simulink model "example_Storage_type3conf"  (R2016b)
settings: Solver=ode45  StartTime=0.0  StopTime=3*3600-2  RelTol=1e-3  EnableMultiTasking=on
undefined symbols (not defined in the file): path_carnot
libraries: carnot x12, simulink x3
settings Model: Creator=drhf  LastModifiedBy=drhf
settings DataIOCC: LimitDataPoints=on  SaveFormat=Array
settings OptimizationCC: ExpressionDepthLimit=2147483647  LifeSpan=inf
settings DebuggingCC: UnderspecifiedInitializationDetection=Classic  MergeDetectMultiDrivingBlocksExec=none  SolverPrmCheckMsg=warning  StateNameClashWarn=warning  SFUnexpectedBacktrackingDiag=warning  SFNoUnconditionalDefaultTransitionDiag=warning  SFExecutionAtInitializationDiag=none
settings HardwareCC: ProdBitPerPointer=32  ProdBitPerSizeT=32  ProdBitPerPtrDiffT=32  ProdLargestAtomicFloat=None  ProdIntDivRoundTo=Undefined  ProdEndianess=Unspecified  ProdWordSize=32  ProdHWDeviceType=32-bit Generic
settings ModelReferenceCC: PropagateSignalLabelsOutOfModel=off
settings GRTTargetCC: TargetLangStandard=C89/C90 (ANSI)  GeneratePreprocessorConditionals=Disable all  CombineOutputUpdateFcns=off  GRTInterface=on
settings ConfigComp: CovMetricSettings=dw  CovHtmlReporting=on  CovSaveCumulativeToWorkspaceVar=on  CovSaveSingleToWorkspaceVar=on  CovExternalEMLEnable=off

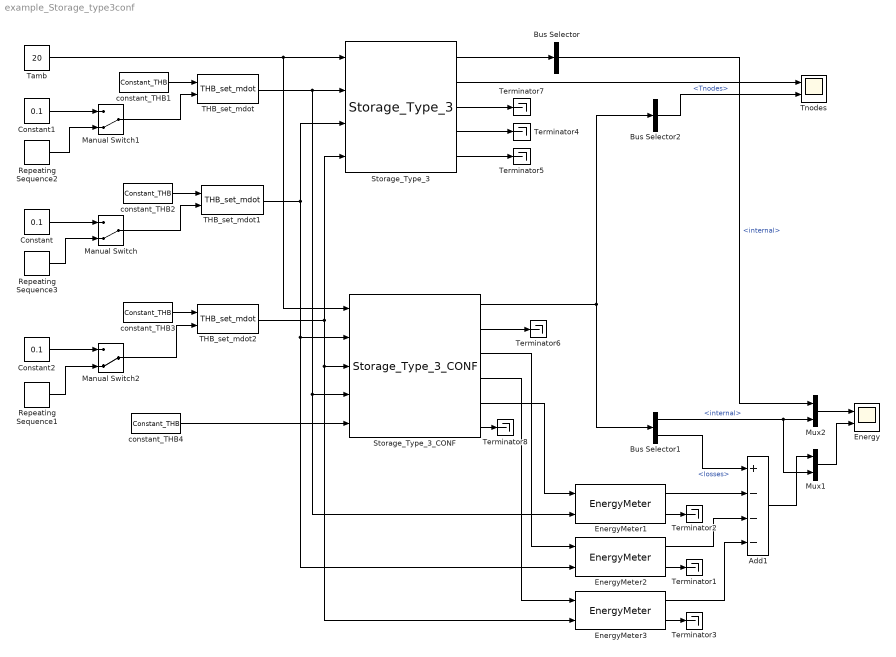
== system example_Storage_type3conf ==
  Add1 : Sum  Inputs=+---
  Bus Selector : BusSelector  OutputSignals=energy.internal
  Bus Selector1 : BusSelector  OutputSignals=energy.internal,energy.losses
  Bus Selector2 : BusSelector  OutputSignals=Tnodes
  Constant : Constant  Value=0.1
  Constant1 : Constant  Value=0.1
  Constant2 : Constant  Value=0.1
  Energy : Scope  NumInputPorts=2
  EnergyMeter1 : carnot/Control/EnergyMeter
  EnergyMeter2 : carnot/Control/EnergyMeter
  EnergyMeter3 : carnot/Control/EnergyMeter
  Manual Switch : ManualSwitch  CurrentSetting=0
  Manual Switch1 : ManualSwitch  CurrentSetting=0
  Manual Switch2 : ManualSwitch  CurrentSetting=0
  Mux1 : Mux  Inputs=2
  Mux2 : Mux  Inputs=2
  Repeating Sequence1 : simulink/Sources/Repeating Sequence  rep_seq_t=[ 0 3600 3600+eps(3600) 7200 7200+eps(7200) 10800]  rep_seq_y=[ 0.12 0.12 0.11+0*eps(3600) 0.11 0.05+0*eps(7200) 0.05]
  Repeating Sequence2 : simulink/Sources/Repeating Sequence  rep_seq_t=[ 0 3600 3600+eps(3600) 7200 7200+eps(7200) 10440 10440+eps(10440) 11160]  rep_seq_y=[ 0 0 0.05+0*eps(3600) 0.05 0.2+0*eps(7200) 0.2 0+0*eps(10440) 0]
  Repeating Sequence3 : simulink/Sources/Repeating Sequence  rep_seq_t=[ 0 3600 3600+eps(3600) 7200 7200+eps(7200) 10800]  rep_seq_y=[ 0 0 0.1+0*eps(3600) 0.1 0.15+0*eps(7200) 0.15]
  Storage_Type_3 : carnot/Storage/Thermal/Storage_Type_3  uloss=1  ubot=1  utop=1  cond=1  volume=0.3  dia=0.5  pos=standing cylinder  h_in_hxup=0.81  h_out_hxup=0.56  ua0_hxup=80  uam_hxup=0.2  uat_hxup=0.5  dplin_hxup=100  dpqua_hxup=100  h_in_hxlw=0.48  h_out_hxlw=0.04  ua0_hxlw=100  uam_hxlw=0.2  uat_hxlw=0.5  dplin_hxlw=100  dpqua_hxlw=100  h_in=0  h_out=1  diapipe=0.04  t0=[10:5:55]  nodes=10  mpoints=10
  Storage_Type_3_CONF : carnot/Storage/Thermal/Storage_Type_3_CONF  t0=[10:5:55]  hgt=1.5279  stgtype=3  tini=[10 15 20 25 30 35 40 45 50 55]  mpts=[1 2 3 4 5 6 7 8 9 10]  PathName=fullfile(path_carnot('libsl'),'Storage','Thermal','Storage_Type_3_CONF','parameter_set')  FileName='StorageType3_300_L.mat'  userPath=off  userParam=off  uwall=1  ubot=1  utop=1  axcond=1  volume=0.3  dia=0.5  standing=standing cylinder  nodes=10  mpoints=10  Tsensor=[0.1 0.5 0.7]  hx1inlet=0.8  hx1outlet=0.6  hx1dia=0.03  hx1uac=50  hx1uam=0.15  hx1uat=0.6  hx1dpqua=20  hx1dplin=20  hx2inlet=0.4  hx2outlet=0  hx2dia=0.03  hx2uac=100  hx2uam=0.15  hx2uat=0.6  hx2dplin=30  hx2dpqua=30  pipe1inlet=0  pipe1outlet=1  pipe1dia=0.03  pipe2inlet=0.6  pipe2outlet=1  pipe2dia=0.03
  THB_set_mdot : carnot/Source/Simple/THB_set_mdot
  THB_set_mdot1 : carnot/Source/Simple/THB_set_mdot
  THB_set_mdot2 : carnot/Source/Simple/THB_set_mdot
  Tamb : Constant  Value=20
  Terminator{1..8} (8 alike) : Terminator
  Tnodes : Scope  NumInputPorts=2
  constant_THB1 : carnot/Source/Simple/Constant_THB  t=10  mdot=0*100/3600  p=1e5  mID=Full Pressure Drop with Static Height  fluid=Water  mix=0  mix2=0  mix3=0  dia=0.02  hgt=0
  constant_THB2 : carnot/Source/Simple/Constant_THB  t=55  mdot=0*100/3600  p=1e5  mID=Full Pressure Drop with Static Height  fluid=Water  mix=0  mix2=0  mix3=0  dia=0.02  hgt=0
  constant_THB3 : carnot/Source/Simple/Constant_THB  t=35  mdot=0*100/3600  p=1e5  mID=Full Pressure Drop with Static Height  fluid=Water  mix=0  mix2=0  mix3=0  dia=0.02  hgt=0
  constant_THB4 : carnot/Source/Simple/Constant_THB  t=35  mdot=0  p=1e5  mID=Full Pressure Drop with Static Height  fluid=Water  mix=0  mix2=0  mix3=0  dia=0.02  hgt=0
  wires:
  Bus Selector/1 -> Mux2/1  "<internal>"
  Tamb/1 -> Storage_Type_3_CONF/1, Storage_Type_3/1
  THB_set_mdot/1 -> Storage_Type_3/2, Storage_Type_3_CONF/4, EnergyMeter1/2
  THB_set_mdot1/1 -> Storage_Type_3/3, Storage_Type_3_CONF/2, EnergyMeter2/2
  Storage_Type_3/1 -> Bus Selector/1
  EnergyMeter2/2 -> Terminator1/1
  Manual Switch1/1 -> THB_set_mdot/2
  Manual Switch/1 -> THB_set_mdot1/2
  Constant/1 -> Manual Switch/1
  Repeating Sequence3/1 -> Manual Switch/2
  Constant1/1 -> Manual Switch1/1
  Repeating Sequence2/1 -> Manual Switch1/2
  EnergyMeter1/2 -> Terminator2/1
  Add1/1 -> Mux1/1
  EnergyMeter2/1 -> Add1/3
  EnergyMeter1/1 -> Add1/2
  Manual Switch2/1 -> THB_set_mdot2/2
  Constant2/1 -> Manual Switch2/1
  Repeating Sequence1/1 -> Manual Switch2/2
  THB_set_mdot2/1 -> Storage_Type_3_CONF/3, EnergyMeter3/2, Storage_Type_3/4
  Storage_Type_3/2 -> Tnodes/1
  EnergyMeter3/2 -> Terminator3/1
  EnergyMeter3/1 -> Add1/4
  constant_THB1/1 -> THB_set_mdot/1
  constant_THB2/1 -> THB_set_mdot1/1
  constant_THB3/1 -> THB_set_mdot2/1
  Storage_Type_3_CONF/1 -> Bus Selector1/1, Bus Selector2/1
  Bus Selector1/1 -> Mux2/2, Mux1/2  "<internal>"
  Bus Selector2/1 -> Tnodes/2  "<Tnodes>"
  Storage_Type_3_CONF/2 -> Terminator6/1
  constant_THB4/1 -> Storage_Type_3_CONF/5
  Storage_Type_3/3 -> Terminator7/1
  Storage_Type_3/4 -> Terminator4/1
  Storage_Type_3/5 -> Terminator5/1
  Mux2/1 -> Energy/1
  Mux1/1 -> Energy/2
  Storage_Type_3_CONF/6 -> Terminator8/1
  Storage_Type_3_CONF/3 -> EnergyMeter2/1
  Storage_Type_3_CONF/5 -> EnergyMeter1/1
  Storage_Type_3_CONF/4 -> EnergyMeter3/1
  Bus Selector1/2 -> Add1/1  "<losses>"
